simulink library "INT_RailP_DD1ms"  (R2016b)
settings: Solver=VariableStepAuto  StartTime=0.0  StopTime=10.0  RelTol=1e-3
settings Model: Creator=zhoutinglin  LastModifiedBy=zhoutinglin

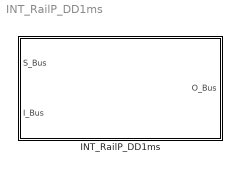
== system INT_RailP_DD1ms ==
  INT_RailP_DD1ms : Subsystem

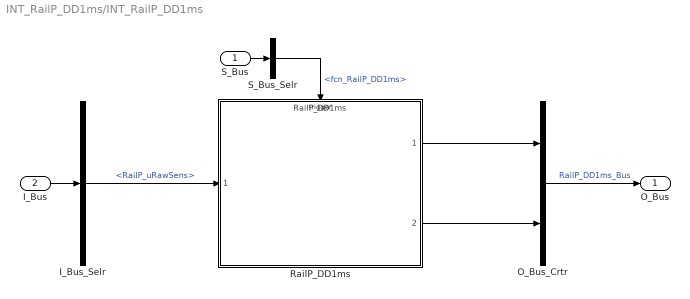
== system INT_RailP_DD1ms/INT_RailP_DD1ms ==
  S_Bus : Inport
  I_Bus : Inport  Port=2
  I_Bus_Selr : BusSelector  OutputSignals=RailP_uRawSens
  O_Bus_Crtr : BusCreator  Inputs=2
  RailP_DD1ms : ModelReference  ModelNameDialog=RailP_DD1ms  SimulationMode=Normal  ModelReferenceVersion=1.6  TriggerPortName=function  TriggerPortTriggerType=function-call  TriggerPortStatesWhenEnabling=held
  S_Bus_Selr : BusSelector  OutputSignals=fcn_RailP_DD1ms
  O_Bus : Outport
  wires:
  S_Bus_Selr/1 -> RailP_DD1ms/Trigger  "<fcn_RailP_DD1ms>"
  S_Bus/1 -> S_Bus_Selr/1
  I_Bus/1 -> I_Bus_Selr/1
  I_Bus_Selr/1 -> RailP_DD1ms/1  "<RailP_uRawSens>"
  O_Bus_Crtr/1 -> O_Bus/1  "RailP_DD1ms_Bus"
  RailP_DD1ms/1 -> O_Bus_Crtr/1
  RailP_DD1ms/2 -> O_Bus_Crtr/2
